simulink model "Example1_7"  (Simulink 7.7)
settings: Solver=ode45  StartTime=0.0  StopTime=T  MaxStep=MaxStep  RelTol=RelTol
values from neighbouring files (symbols this model uses):
  J = 15    [initialization_ex1_7.m]
  rule = 1    [initialization_ex1_7.m]
  T = 15    [initialization_ex1_7.m]
  x1_0 = 0.5    [ex1_7_v3_0_0.m]    (also in initialization_ex1_7.m = [0.5])
  x2_0 = 0    [ex1_7_v3_0_0.m]    (also in initialization_ex1_7.m = [0])
libraries: simulink x6
settings Model: Creator=pablonanez  LastModifiedBy=pablonanez
settings SFSimCC: SimParseCustomCode=off

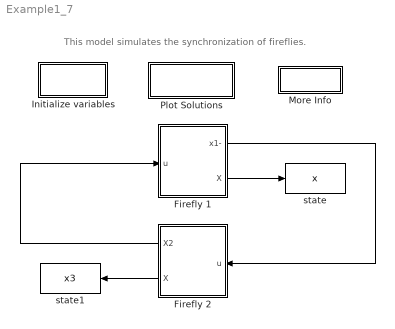
== system Example1_7 ==
  note: This model simulates the synchronization of fireflies.
  Firefly 1 : Subsystem  LoadFcn=set_param(gcb,'LinkStatus','none')
      settings: CopyFcn=|
      | set_param(gcb,'LinkStatus','none')
      | set_param(gcs, 'MaxStep', 'MaxStep', 'RelTol', 'RelTol')
      mask Display:
      | image(imread('Hcal.jpg'))
      | %plot([5 20 20 5 5],[5 5 20 20 5])
      | %text(8,13,'HyEq_mdl')
      | port_label('output', 1, 'x-')
      | port_label('input', 1, 'u')
  Firefly 2 : Subsystem  LoadFcn=set_param(gcb,'LinkStatus','none')
      settings: CopyFcn=|
      | set_param(gcb,'LinkStatus','none')
      | set_param(gcs, 'MaxStep', 'MaxStep', 'RelTol', 'RelTol')
      mask Display:
      | image(imread('Hcal.jpg'))
      | %plot([5 20 20 5 5],[5 5 20 20 5])
      | %text(8,13,'HyEq_mdl')
      | port_label('output', 1, 'x-')
      | port_label('input', 1, 'u')
  Initialize variables : Subsystem  Priority=-10
      settings: OpenFcn=initialization_ex1_7
      mask Display: disp('Double Click\n to Initialize')
  More Info : Subsystem
      settings: OpenFcn=helpview 'Example_1_7.html'
      mask Display: disp('More Info')
  Plot Solutions : Subsystem
      settings: OpenFcn=postprocessing_ex1_7
      mask Display: disp('Double Click to\n Plot Solutions')
  state : ToWorkspace  VariableName=x  SampleTime=-1  SaveFormat=Array
  state1 : ToWorkspace  VariableName=x3  SampleTime=-1  SaveFormat=Array
  wires:
  Firefly 1/1(x1-) -> Firefly 2/1(u)
  Firefly 2/1(X2) -> Firefly 1/1(u)
  Firefly 1/2(X) -> state/1
  Firefly 2/2(X) -> state1/1

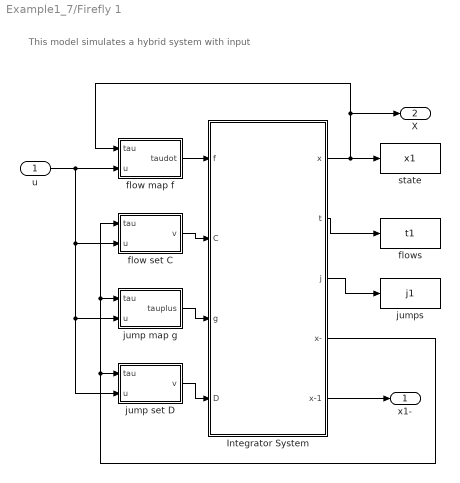
== system Example1_7/Firefly 1 ==
  note: This model simulates a hybrid system with input
  u : Inport
  Integrator System : Subsystem  Priority=2  mask(Hybrid Integrator){T=T, J=J, x0=x1_0}
      mask prompts: T "Flow Horizon"; J "Jump Horizon"; x0 "Initial Condition"
      mask help:
      | This block integrates the state of the hybrid system defined by the flow map f (first input), the flow set C (second input), the jump map g (third input) and the jump set D (fourth input).
      | Starting from the initial condition x0 (last mask parameter), the system's state x evolves continuously within the set C, according to f(x,u), but is also subject to jumps within D, according to g(x,u).
      | The block also stops the simulation when the time t is greater than the flow horizon T (first mask parameter), or when the number of jumps j is greater than the jump horizon J (second mask parameter).
      | The outputs of the blocks are respectively x(t), t, j, x(t-).
      mask Help:
      | This block integrates the state of the hybrid system defined by the flow map f (first input), the flow set C (second input), the jump map g (third input) and the jump set D (fourth input).
      | <br>
      | Starting from the initial condition x0 (last mask parameter), the system's state x evolves continuously within the set C, according to f(x,u), but is also subject to jumps within D, according to g(x,u).
      | <br>
      | The block also stops the simulation when the time t is greater than the flow horizon T (first mask parameter), or when the number of jumps j is greater than the jump horizon J (second mask parameter).
      | <br>
      | The outputs of the blocks are respectively x(t), t, j, x(t-).
      | <br>
      | You can right click on the block and "Look under mask" to see what's inside the block.
      | Finally, refer to the manual (HybridSimulator_vXX.pdf) for more detailed information on how this hybrid simulator works.
  flow map f : Stateflow chart  TreatAsAtomicUnit=on
  flow set C : Stateflow chart  TreatAsAtomicUnit=on
  flows : ToWorkspace  VariableName=t1  SampleTime=-1  SaveFormat=Array
  jump map g : Stateflow chart  Priority=2  TreatAsAtomicUnit=on
  jump set D : Stateflow chart  TreatAsAtomicUnit=on
  jumps : ToWorkspace  VariableName=j1  SampleTime=-1  SaveFormat=Array
  state : ToWorkspace  VariableName=x1  SampleTime=-1  SaveFormat=Array
  x1- : Outport
  X : Outport  Port=2
  wires:
  jump map g/1(tauplus) -> Integrator System/3(g)
  jump set D/1(v) -> Integrator System/4(D)
  u/1 -> jump set D/2(u), jump map g/2(u), flow set C/2(u), flow map f/2(u)
  flow set C/1(v) -> Integrator System/2(C)
  flow map f/1(taudot) -> Integrator System/1(f)
  Integrator System/1(x) -> state/1, flow map f/1(tau), X/1
  Integrator System/2(t) -> flows/1
  Integrator System/3(j) -> jumps/1
  Integrator System/4(x-) -> jump set D/1(tau), jump map g/1(tau), flow set C/1(tau)
  Integrator System/5(x-1) -> x1-/1

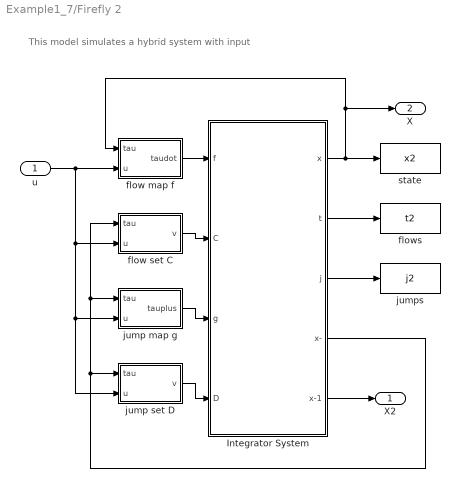
== system Example1_7/Firefly 2 ==
  note: This model simulates a hybrid system with input
  u : Inport
  Integrator System : Subsystem  Priority=2  mask(Hybrid Integrator){T=T, J=J, x0=x2_0}
      mask prompts: T "Flow Horizon"; J "Jump Horizon"; x0 "Initial Condition"
      mask help:
      | This block integrates the state of the hybrid system defined by the flow map f (first input), the flow set C (second input), the jump map g (third input) and the jump set D (fourth input).
      | Starting from the initial condition x0 (last mask parameter), the system's state x evolves continuously within the set C, according to f(x,u), but is also subject to jumps within D, according to g(x,u).
      | The block also stops the simulation when the time t is greater than the flow horizon T (first mask parameter), or when the number of jumps j is greater than the jump horizon J (second mask parameter).
      | The outputs of the blocks are respectively x(t), t, j, x(t-).
      mask Help:
      | This block integrates the state of the hybrid system defined by the flow map f (first input), the flow set C (second input), the jump map g (third input) and the jump set D (fourth input).
      | <br>
      | Starting from the initial condition x0 (last mask parameter), the system's state x evolves continuously within the set C, according to f(x,u), but is also subject to jumps within D, according to g(x,u).
      | <br>
      | The block also stops the simulation when the time t is greater than the flow horizon T (first mask parameter), or when the number of jumps j is greater than the jump horizon J (second mask parameter).
      | <br>
      | The outputs of the blocks are respectively x(t), t, j, x(t-).
      | <br>
      | You can right click on the block and "Look under mask" to see what's inside the block.
      | Finally, refer to the manual (HybridSimulator_vXX.pdf) for more detailed information on how this hybrid simulator works.
  flow map f : Stateflow chart  TreatAsAtomicUnit=on
  flow set C : Stateflow chart  TreatAsAtomicUnit=on
  flows : ToWorkspace  VariableName=t2  SampleTime=-1  SaveFormat=Array
  jump map g : Stateflow chart  Priority=2  TreatAsAtomicUnit=on
  jump set D : Stateflow chart  TreatAsAtomicUnit=on
  jumps : ToWorkspace  VariableName=j2  SampleTime=-1  SaveFormat=Array
  state : ToWorkspace  VariableName=x2  SampleTime=-1  SaveFormat=Array
  X2 : Outport
  X : Outport  Port=2
  wires:
  jump map g/1(tauplus) -> Integrator System/3(g)
  jump set D/1(v) -> Integrator System/4(D)
  u/1 -> jump set D/2(u), jump map g/2(u), flow set C/2(u), flow map f/2(u)
  flow set C/1(v) -> Integrator System/2(C)
  flow map f/1(taudot) -> Integrator System/1(f)
  Integrator System/1(x) -> state/1, flow map f/1(tau), X/1
  Integrator System/2(t) -> flows/1
  Integrator System/3(j) -> jumps/1
  Integrator System/5(x-1) -> X2/1
  Integrator System/4(x-) -> jump set D/1(tau), jump map g/1(tau), flow set C/1(tau)

== system Example1_7/Initialize variables ==

== system Example1_7/More Info ==

== system Example1_7/Plot Solutions ==

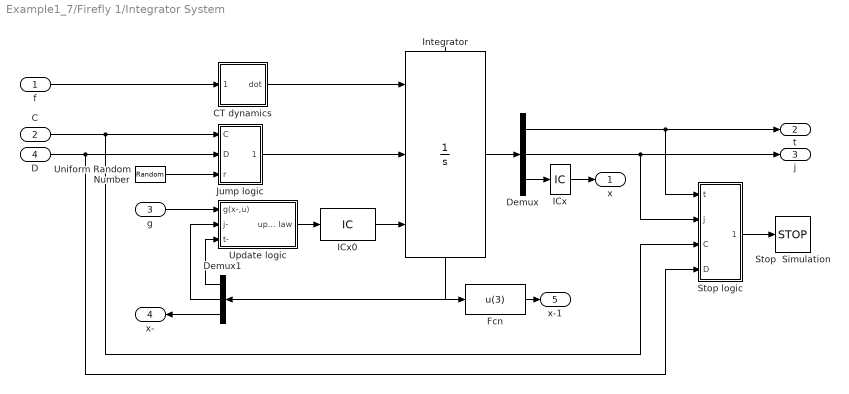
== system Example1_7/Firefly 1/Integrator System ==
  f : Inport
  C : Inport  Port=2
  g : Inport  Port=3
  D : Inport  Port=4
  CT dynamics : Subsystem
  Demux : Demux  Outputs=[1 1 -1]
  Demux1 : Demux  Outputs=[1 1 -1]
  Fcn : Fcn  Expr=u(3)
  ICx : InitialCondition  Value=x0
  ICx0 : InitialCondition  Value=[0; 0; x0(:)]
  Integrator : Integrator  ExternalReset=level hold  InitialConditionSource=external  ShowStatePort=on  ZeroCross=off
  Jump logic : Subsystem
  Stop  Simulation : Stop
  Stop logic : Subsystem
  Uniform Random Number : UniformRandomNumber  Minimum=0  Seed=abs(floor(100*rand))  SampleTime=0
  Update logic : Subsystem
  x : Outport
  t : Outport  Port=2
  j : Outport  Port=3
  x- : Outport  Port=4
  x-1 : Outport  Port=5
  wires:
  Demux1/2 -> Update logic/2(j-)
  Demux1/1 -> Update logic/3(t-)
  g/1 -> Update logic/1(g(x-,u))
  Uniform Random Number/1 -> Jump logic/3(r)
  Jump logic/1(jump) -> Integrator/2
  f/1 -> CT dynamics/1(f(x,u))
  D/1 -> Jump logic/2(D), Stop logic/4(D)
  C/1 -> Jump logic/1(C), Stop logic/3(C)
  Integrator/1 -> Demux/1
  Stop logic/1(stop) -> Stop  Simulation/1
  CT dynamics/1(dot) -> Integrator/1
  Update logic/1(update law) -> ICx0/1
  Demux/1 -> Stop logic/1(t), t/1
  Demux/2 -> Stop logic/2(j), j/1
  Integrator/State -> Demux1/1, Fcn/1
  Demux/3 -> ICx/1
  ICx/1 -> x/1
  ICx0/1 -> Integrator/3
  Demux1/3 -> x-/1
  Fcn/1 -> x-1/1

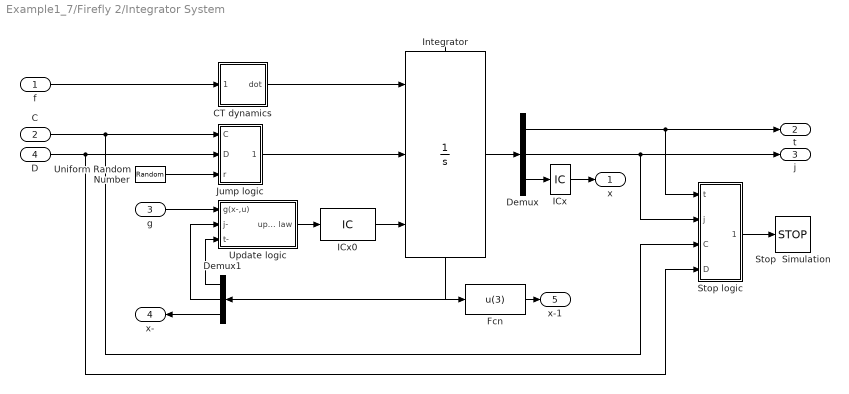
== system Example1_7/Firefly 2/Integrator System ==
  f : Inport
  C : Inport  Port=2
  g : Inport  Port=3
  D : Inport  Port=4
  CT dynamics : Subsystem
  Demux : Demux  Outputs=[1 1 -1]
  Demux1 : Demux  Outputs=[1 1 -1]
  Fcn : Fcn  Expr=u(3)
  ICx : InitialCondition  Value=x0
  ICx0 : InitialCondition  Value=[0; 0; x0(:)]
  Integrator : Integrator  ExternalReset=level hold  InitialConditionSource=external  ShowStatePort=on  ZeroCross=off
  Jump logic : Subsystem
  Stop  Simulation : Stop
  Stop logic : Subsystem
  Uniform Random Number : UniformRandomNumber  Minimum=0  Seed=abs(floor(100*rand))  SampleTime=0
  Update logic : Subsystem
  x : Outport
  t : Outport  Port=2
  j : Outport  Port=3
  x- : Outport  Port=4
  x-1 : Outport  Port=5
  wires:
  Demux1/2 -> Update logic/2(j-)
  Demux1/1 -> Update logic/3(t-)
  g/1 -> Update logic/1(g(x-,u))
  Uniform Random Number/1 -> Jump logic/3(r)
  Jump logic/1(jump) -> Integrator/2
  f/1 -> CT dynamics/1(f(x,u))
  D/1 -> Jump logic/2(D), Stop logic/4(D)
  C/1 -> Jump logic/1(C), Stop logic/3(C)
  Integrator/1 -> Demux/1
  Stop logic/1(stop) -> Stop  Simulation/1
  CT dynamics/1(dot) -> Integrator/1
  Update logic/1(update law) -> ICx0/1
  Demux/1 -> Stop logic/1(t), t/1
  Demux/2 -> Stop logic/2(j), j/1
  Integrator/State -> Demux1/1, Fcn/1
  Demux/3 -> ICx/1
  ICx/1 -> x/1
  ICx0/1 -> Integrator/3
  Demux1/3 -> x-/1
  Fcn/1 -> x-1/1

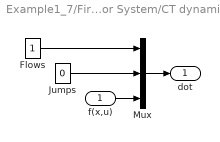
== system Example1_7/Firefly 1/Integrator System/CT dynamics ==
  f(x,u) : Inport
  Flows : Constant
  Jumps : Constant  Value=0
  Mux : Mux  Inputs=[1 1 -1]
  dot : Outport
  wires:
  f(x,u)/1 -> Mux/3
  Mux/1 -> dot/1
  Flows/1 -> Mux/1
  Jumps/1 -> Mux/2

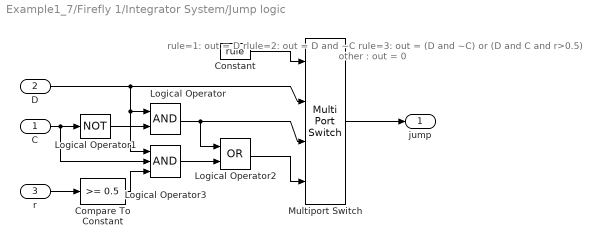
== system Example1_7/Firefly 1/Integrator System/Jump logic ==
  note: rule=1:  out = D
      | rlule=2: out = D and ~C
      | rule=3:  out = (D and ~C)  or (D and C and r>0.5)
      | other :  out = 0
  C : Inport
  D : Inport  Port=2
  r : Inport  Port=3
  Compare To Constant : simulink/Logic and Bit Operations/Compare To Constant  SystemSampleTime=-1  relop=>=  const=0.5  LogicOutDataTypeMode=uint8
  Constant : Constant  Value=rule
  Logical Operator : Logic  AllPortsSameDT=off  OutDataTypeStr=boolean
  Logical Operator1 : Logic  Operator=NOT  Inputs=1  AllPortsSameDT=off  OutDataTypeStr=boolean
  Logical Operator2 : Logic  Operator=OR  AllPortsSameDT=off  OutDataTypeStr=boolean
  Logical Operator3 : Logic  Inputs=3  AllPortsSameDT=off  OutDataTypeStr=boolean
  Multiport Switch : MultiPortSwitch  zeroidx=off
  jump : Outport
  wires:
  Logical Operator3/1 -> Logical Operator2/2
  Compare To Constant/1 -> Logical Operator3/3
  Multiport Switch/1 -> jump/1
  Logical Operator2/1 -> Multiport Switch/4
  Logical Operator/1 -> Logical Operator2/1, Multiport Switch/3
  Logical Operator1/1 -> Logical Operator/2
  C/1 -> Logical Operator1/1, Logical Operator3/2
  r/1 -> Compare To Constant/1
  D/1 -> Multiport Switch/2, Logical Operator/1, Logical Operator3/1
  Constant/1 -> Multiport Switch/1

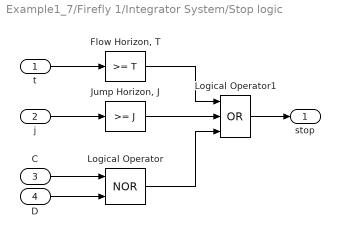
== system Example1_7/Firefly 1/Integrator System/Stop logic ==
  t : Inport
  j : Inport  Port=2
  C : Inport  Port=3
  D : Inport  Port=4
  "Flow Horizon, T" : simulink/Logic and Bit Operations/Compare To Constant  SystemSampleTime=-1  relop=>=  const=T  LogicOutDataTypeMode=uint8  ZeroCross=off
  "Jump Horizon, J" : simulink/Logic and Bit Operations/Compare To Constant  SystemSampleTime=-1  relop=>=  const=J  LogicOutDataTypeMode=uint8  ZeroCross=off
  Logical Operator : Logic  Operator=NOR  AllPortsSameDT=off  OutDataTypeStr=boolean
  Logical Operator1 : Logic  Operator=OR  Inputs=3  AllPortsSameDT=off  OutDataTypeStr=boolean
  stop : Outport
  wires:
  Logical Operator1/1 -> stop/1
  C/1 -> Logical Operator/1
  j/1 -> "Jump Horizon, J"/1
  t/1 -> "Flow Horizon, T"/1
  D/1 -> Logical Operator/2
  Logical Operator/1 -> Logical Operator1/3
  "Jump Horizon, J"/1 -> Logical Operator1/2
  "Flow Horizon, T"/1 -> Logical Operator1/1

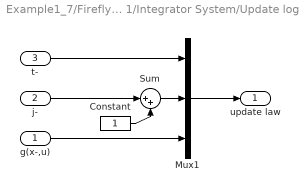
== system Example1_7/Firefly 1/Integrator System/Update logic ==
  g(x-,u) : Inport
  j- : Inport  Port=2
  t- : Inport  Port=3
  Constant : Constant
  Mux1 : Mux  Inputs=[1 1 -1]
  Sum : Sum  Inputs=|++
  update law : Outport
  wires:
  Constant/1 -> Sum/2
  t-/1 -> Mux1/1
  g(x-,u)/1 -> Mux1/3
  j-/1 -> Sum/1
  Mux1/1 -> update law/1
  Sum/1 -> Mux1/2

== system Example1_7/Firefly 2/Integrator System/CT dynamics ==
  f(x,u) : Inport
  Flows : Constant
  Jumps : Constant  Value=0
  Mux : Mux  Inputs=[1 1 -1]
  dot : Outport
  wires:
  f(x,u)/1 -> Mux/3
  Mux/1 -> dot/1
  Flows/1 -> Mux/1
  Jumps/1 -> Mux/2

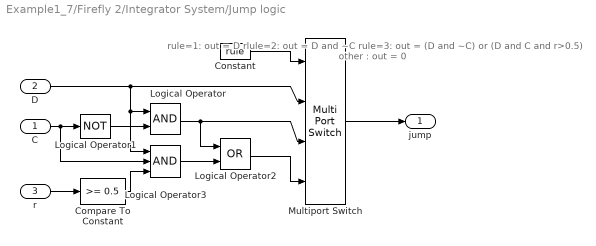
== system Example1_7/Firefly 2/Integrator System/Jump logic ==
  note: rule=1:  out = D
      | rlule=2: out = D and ~C
      | rule=3:  out = (D and ~C)  or (D and C and r>0.5)
      | other :  out = 0
  C : Inport
  D : Inport  Port=2
  r : Inport  Port=3
  Compare To Constant : simulink/Logic and Bit Operations/Compare To Constant  SystemSampleTime=-1  relop=>=  const=0.5  LogicOutDataTypeMode=uint8
  Constant : Constant  Value=rule
  Logical Operator : Logic  AllPortsSameDT=off  OutDataTypeStr=boolean
  Logical Operator1 : Logic  Operator=NOT  Inputs=1  AllPortsSameDT=off  OutDataTypeStr=boolean
  Logical Operator2 : Logic  Operator=OR  AllPortsSameDT=off  OutDataTypeStr=boolean
  Logical Operator3 : Logic  Inputs=3  AllPortsSameDT=off  OutDataTypeStr=boolean
  Multiport Switch : MultiPortSwitch  zeroidx=off
  jump : Outport
  wires:
  Logical Operator3/1 -> Logical Operator2/2
  Compare To Constant/1 -> Logical Operator3/3
  Multiport Switch/1 -> jump/1
  Logical Operator2/1 -> Multiport Switch/4
  Logical Operator/1 -> Logical Operator2/1, Multiport Switch/3
  Logical Operator1/1 -> Logical Operator/2
  C/1 -> Logical Operator1/1, Logical Operator3/2
  r/1 -> Compare To Constant/1
  D/1 -> Multiport Switch/2, Logical Operator/1, Logical Operator3/1
  Constant/1 -> Multiport Switch/1

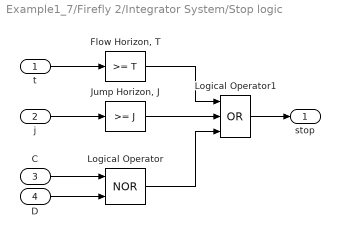
== system Example1_7/Firefly 2/Integrator System/Stop logic ==
  t : Inport
  j : Inport  Port=2
  C : Inport  Port=3
  D : Inport  Port=4
  "Flow Horizon, T" : simulink/Logic and Bit Operations/Compare To Constant  SystemSampleTime=-1  relop=>=  const=T  LogicOutDataTypeMode=uint8  ZeroCross=off
  "Jump Horizon, J" : simulink/Logic and Bit Operations/Compare To Constant  SystemSampleTime=-1  relop=>=  const=J  LogicOutDataTypeMode=uint8  ZeroCross=off
  Logical Operator : Logic  Operator=NOR  AllPortsSameDT=off  OutDataTypeStr=boolean
  Logical Operator1 : Logic  Operator=OR  Inputs=3  AllPortsSameDT=off  OutDataTypeStr=boolean
  stop : Outport
  wires:
  Logical Operator1/1 -> stop/1
  C/1 -> Logical Operator/1
  j/1 -> "Jump Horizon, J"/1
  t/1 -> "Flow Horizon, T"/1
  D/1 -> Logical Operator/2
  Logical Operator/1 -> Logical Operator1/3
  "Jump Horizon, J"/1 -> Logical Operator1/2
  "Flow Horizon, T"/1 -> Logical Operator1/1

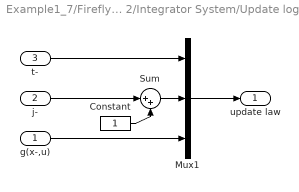
== system Example1_7/Firefly 2/Integrator System/Update logic ==
  g(x-,u) : Inport
  j- : Inport  Port=2
  t- : Inport  Port=3
  Constant : Constant
  Mux1 : Mux  Inputs=[1 1 -1]
  Sum : Sum  Inputs=|++
  update law : Outport
  wires:
  Constant/1 -> Sum/2
  t-/1 -> Mux1/1
  g(x-,u)/1 -> Mux1/3
  j-/1 -> Sum/1
  Mux1/1 -> update law/1
  Sum/1 -> Mux1/2

== matlab function Firefly 1/flow map f ==
  data: tau input double; taudot output double; u input double
function taudot = f(tau, u)

%%%%%%%%%%%%%%%%%%%%%%%%%%%%%%%%%%%%%%%%%%%%%%%%%%%%%%%%%%%%%%%%%%%%%%%%%%%
% Matlab Function  Author: Ricardo Sanfelice
%
% Project: Simulation of a hybrid system (interconnection)
%
% Name: f.m
%
% Description: Flow map
%
% Version: 1.0
% Required files: - 
%%%%%%%%%%%%%%%%%%%%%%%%%%%%%%%%%%%%%%%%%%%%%%%%%%%%%%%%%%%%%%%%%%%%%%%%%%%

% flow map
taudot = 1;

== matlab function Firefly 1/flow set C ==
  data: tau input double; v output double; u input double
function v  = C(tau, u) 

%%%%%%%%%%%%%%%%%%%%%%%%%%%%%%%%%%%%%%%%%%%%%%%%%%%%%%%%%%%%%%%%%%%%%%%%%%%
% Matlab Function  Author: Ricardo Sanfelice 
%
% Project: Simulation of a hybrid system (interconnection)
%
% Name: C.m
%
% Description: Flow set
%
% Version: 1.0
% Required files: - 
%%%%%%%%%%%%%%%%%%%%%%%%%%%%%%%%%%%%%%%%%%%%%%%%%%%%%%%%%%%%%%%%%%%%%%%%%%%

%flow set
if ((tau > 0) && (tau < 1)) || ((u > 0) && (u <= 1))  % flow condition
    v = 1;  % report flow
else 
    v = 0;  % do not report flow
end

== matlab function Firefly 2/flow map f ==
  data: tau input double; taudot output double; u input double
function taudot = f(tau, u)

%%%%%%%%%%%%%%%%%%%%%%%%%%%%%%%%%%%%%%%%%%%%%%%%%%%%%%%%%%%%%%%%%%%%%%%%%%%
% Matlab Function  Author: Ricardo Sanfelice
%
% Project: Simulation of a hybrid system (interconnection)
%
% Name: f.m
%
% Description: Flow map
%
% Version: 1.0
% Required files: - 
%%%%%%%%%%%%%%%%%%%%%%%%%%%%%%%%%%%%%%%%%%%%%%%%%%%%%%%%%%%%%%%%%%%%%%%%%%%

% flow map
taudot = 1;

== matlab function Firefly 2/flow set C ==
  data: tau input double; v output double; u input double
function v  = C(tau, u) 

%%%%%%%%%%%%%%%%%%%%%%%%%%%%%%%%%%%%%%%%%%%%%%%%%%%%%%%%%%%%%%%%%%%%%%%%%%%
% Matlab Function  Author: Ricardo Sanfelice 
%
% Project: Simulation of a hybrid system (interconnection)
%
% Name: C.m
%
% Description: Flow set
%
% Version: 1.0
% Required files: - 
%%%%%%%%%%%%%%%%%%%%%%%%%%%%%%%%%%%%%%%%%%%%%%%%%%%%%%%%%%%%%%%%%%%%%%%%%%%

%flow set
if ((tau > 0) && (tau < 1)) || ((u > 0) && (u <= 1))  % flow condition
    v = 1;  % report flow
else 
    v = 0;  % do not report flow
end

== matlab function Firefly 2/jump map g ==
  data: tau input double; tauplus output double; u input double; e parameter double
function tauplus = g(tau, u, e)

%%%%%%%%%%%%%%%%%%%%%%%%%%%%%%%%%%%%%%%%%%%%%%%%%%%%%%%%%%%%%%%%%%%%%%%%%%%
% Matlab Function  Author: Ricardo Sanfelice 
%
% Project: Simulation of a hybrid system (interconnection)
%
% Name: g.m
%
% Description: Jump map
%
% Version: 1.0
% Required files: - 
%%%%%%%%%%%%%%%%%%%%%%%%%%%%%%%%%%%%%%%%%%%%%%%%%%%%%%%%%%%%%%%%%%%%%%%%%%%

% jump map
if (1+e)*tau < 1
    tauplus = (1+e)*tau;
elseif (1+e)*tau >= 1
    tauplus = 0;
else
    tauplus = tau;   
end

== matlab function Firefly 1/jump map g ==
  data: tau input double; tauplus output double; u input double; e parameter double
function tauplus = g(tau, u, e)

%%%%%%%%%%%%%%%%%%%%%%%%%%%%%%%%%%%%%%%%%%%%%%%%%%%%%%%%%%%%%%%%%%%%%%%%%%%
% Matlab Function  Author: Ricardo Sanfelice 
%
% Project: Simulation of a hybrid system (interconnection)
%
% Name: g.m
%
% Description: Jump map
%
% Version: 1.0
% Required files: - 
%%%%%%%%%%%%%%%%%%%%%%%%%%%%%%%%%%%%%%%%%%%%%%%%%%%%%%%%%%%%%%%%%%%%%%%%%%%

% jump map
if (1+e)*tau < 1
    tauplus = (1+e)*tau;
elseif (1+e)*tau >= 1
    tauplus = 0;
else
    tauplus = tau;   
end

== matlab function Firefly 1/jump set D ==
  data: tau input double; v output double; u input double
function v  = D(tau, u) 

%%%%%%%%%%%%%%%%%%%%%%%%%%%%%%%%%%%%%%%%%%%%%%%%%%%%%%%%%%%%%%%%%%%%%%%%%%%
% Matlab Function  Author: Ricardo Sanfelice
%
% Project: Simulation of a hybrid system (interconnection)
%
% Name: D.m
%
% Description: Jump set
%
% Version: 1.0
% Required files: - 
%%%%%%%%%%%%%%%%%%%%%%%%%%%%%%%%%%%%%%%%%%%%%%%%%%%%%%%%%%%%%%%%%%%%%%%%%%%

if (u >= 1) || (tau >= 1) % jump condition
    v = 1;  % report jump
else
    v = 0;  % do not report jump
end

== matlab function Firefly 2/jump set D ==
  data: tau input double; v output double; u input double
function v  = D(tau, u) 

%%%%%%%%%%%%%%%%%%%%%%%%%%%%%%%%%%%%%%%%%%%%%%%%%%%%%%%%%%%%%%%%%%%%%%%%%%%
% Matlab Function  Author: Ricardo Sanfelice
%
% Project: Simulation of a hybrid system (interconnection)
%
% Name: D.m
%
% Description: Jump set
%
% Version: 1.0
% Required files: - 
%%%%%%%%%%%%%%%%%%%%%%%%%%%%%%%%%%%%%%%%%%%%%%%%%%%%%%%%%%%%%%%%%%%%%%%%%%%

if (u >= 1) || (tau >= 1) % jump condition
    v = 1;  % report jump
else
    v = 0;  % do not report jump
end
